simulink model "Speed_Bump_Tests"  (R2023b)
settings: Solver=ode45  StartTime=0.0  StopTime=10  MaxStep=0.01  RelTol=1e-3  EnableMultiTasking=on
settings Model: Creator=acookson  LastModifiedBy=franc
settings SolverCC: AlgebraicLoopSolver=TrustRegion
settings DataIOCC: LimitDataPoints=on  SaveFormat=Array  ReturnWorkspaceOutputs=off
settings OptimizationCC: LifeSpan=inf
settings DebuggingCC: SolverPrmCheckMsg=warning  UnconnectedInputMsg=warning  UnconnectedOutputMsg=warning  UnconnectedLineMsg=warning  SFUnexpectedBacktrackingDiag=warning  SFNoUnconditionalDefaultTransitionDiag=warning  SFExecutionAtInitializationDiag=none  ArithmeticOperatorsInVariantConditions=warning
settings HardwareCC: ProdBitPerPointer=32  ProdBitPerSizeT=32  ProdBitPerPtrDiffT=32  ProdLargestAtomicFloat=None  ProdIntDivRoundTo=Undefined  ProdEndianess=Unspecified  ProdWordSize=32  ProdHWDeviceType=32-bit Generic
settings ModelReferenceCC: EnableRefExpFcnMdlSchedulingChecks=on  PropagateSignalLabelsOutOfModel=off
settings SFSimCC: SimUseLocalCustomCode=off  CustomCodeUndefinedFunction=UseInterfaceOnly
settings RTWCC: RTWUseLocalCustomCode=off
settings CodeAppCC: StateflowObjectComments=on
settings GRTTargetCC: TargetLangStandard=C89/C90 (ANSI)
settings ConfigComp: CovMetricSettings=dw  CovSaveCumulativeToWorkspaceVar=on  CovSaveSingleToWorkspaceVar=on  CovExternalEMLEnable=off  CovSFcnEnable=off

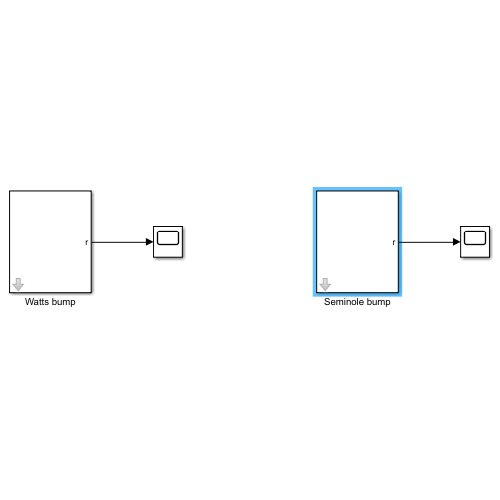
[thumbnail: Simulink's stored preview of the top-level diagram]
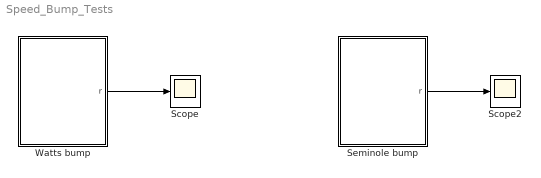
== system Speed_Bump_Tests ==
  Scope : Scope
  Scope2 : Scope
  Seminole bump : Subsystem  mask{h=0.1, d=3, L=6.7, v=8, delta=0, n=4}
      mask prompts: h "Bump height (m)"; d "Top length (m)"; L "Bump length (m)"; v "Vehicle speed (m/s)"; delta "Inter axis (m)"; n "Bump number"
  Watts bump : Subsystem  mask{h=0.1, L=3.7, v=8, delta=0, n=10}
      mask prompts: h "Bump height (m)"; L "Bump length (m)"; v "Vehicle speed (m/s)"; delta "Inter axis (m)"; n "Bump number"
  wires:
  Watts bump/1(r) -> Scope/1
  Seminole bump/1(r) -> Scope2/1

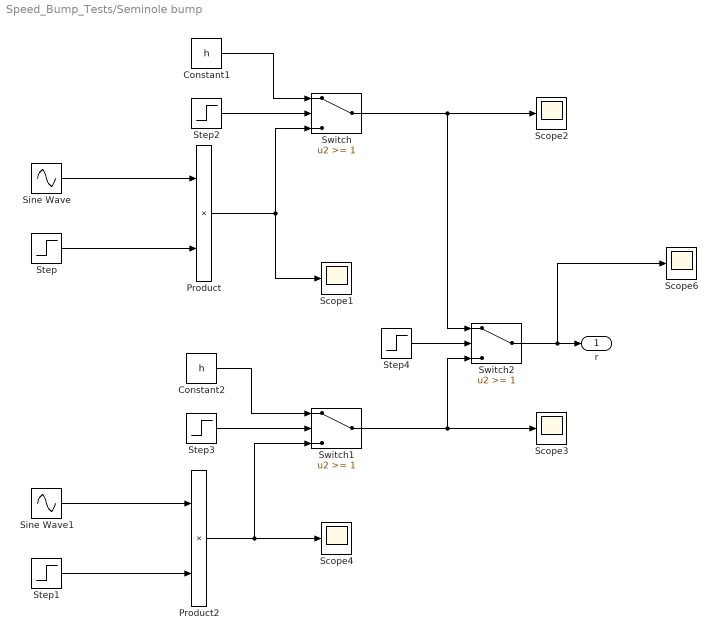
== system Speed_Bump_Tests/Seminole bump ==
  Constant1 : Constant  Value=h
  Constant2 : Constant  Value=h
  Product : Product
  Product2 : Product
  Scope{1..4,6} (5 alike) : Scope
  Sine Wave : Sin  Amplitude=h  Frequency=2*pi*(v/L)  Phase=-2*pi*(delta/L)  SampleTime=0
  Sine Wave1 : Sin  Amplitude=h  Frequency=2*pi*(v/L)  Phase=-2*pi*(delta/L)  SampleTime=0
  Step : Step  Time=n*(L/v)+(delta/v)  SampleTime=0
  Step1 : Step  Time=(n+d+0.5)*(L/v)+(delta/v)  Before=1  After=0  SampleTime=0
  Step2 : Step  Time=(n+0.25)*(L/v)+(delta/v)  SampleTime=0
  Step3 : Step  Time=(n+d+0.25)*(L/v)+(delta/v)  Before=1  After=0  SampleTime=0
  Step4 : Step  Time=(n+d/2+0.25)*(L/v)+(delta/v)  Before=1  After=0  SampleTime=0
  Switch : Switch  Threshold=1  SaturateOnIntegerOverflow=off  InputSameDT=off
  Switch1 : Switch  Threshold=1  SaturateOnIntegerOverflow=off  InputSameDT=off
  Switch2 : Switch  Threshold=1  SaturateOnIntegerOverflow=off  InputSameDT=off
  r : Outport
  wires:
  Sine Wave/1 -> Product/1
  Step/1 -> Product/2
  Switch2/1 -> Scope6/1, r/1
  Step2/1 -> Switch/2
  Constant1/1 -> Switch/1
  Product/1 -> Switch/3, Scope1/1
  Switch/1 -> Switch2/1, Scope2/1
  Sine Wave1/1 -> Product2/1
  Step1/1 -> Product2/2
  Product2/1 -> Scope4/1, Switch1/3
  Constant2/1 -> Switch1/1
  Step3/1 -> Switch1/2
  Switch1/1 -> Scope3/1, Switch2/3
  Step4/1 -> Switch2/2

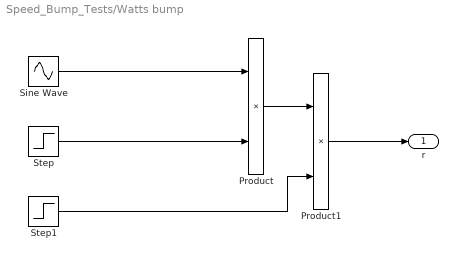
== system Speed_Bump_Tests/Watts bump ==
  Product : Product
  Product1 : Product
  Sine Wave : Sin  Amplitude=h  Frequency=2*pi*(v/L)  Phase=-2*pi*(delta/L)  SampleTime=0
  Step : Step  Time=n*(L/v)+(delta/v)  SampleTime=0
  Step1 : Step  Time=(n+0.5)*(L/v)+(delta/v)  Before=1  After=0  SampleTime=0
  r : Outport
  wires:
  Sine Wave/1 -> Product/1
  Step/1 -> Product/2
  Product/1 -> Product1/1
  Step1/1 -> Product1/2
  Product1/1 -> r/1
